simulink model "ex6_aberta"  (Simulink 8.9)
settings: Solver=FixedStepAuto  StartTime=0.0  StopTime=4  FixedStep=0.00442  RelTol=1e-3  EnableMultiTasking=on
values from neighbouring files (symbols this model uses):
  c1 = 2.94    [exp01e03.m]
  k1 = 338.6    [exp01e03.m]
  khw = 14732    [exp01e03.m]
  kpfA = 1 / Gps0    [exp01e03.m]
  kv = 0.005    [exp01e03.m]
  m1 = mc1 + mw1    (= 2.778)    [exp01e03.m]
settings Model: Creator=Gabriel  LastModifiedBy=Gabriel
settings DataIOCC: LimitDataPoints=off
settings OptimizationCC: InitFltsAndDblsToZero=on
settings DebuggingCC: SaveWithParameterizedLinksMsg=none  SignalResolutionControl=TryResolveAllWithWarning  SolverPrmCheckMsg=warning  MultiTaskDSMMsg=warning  MultiTaskCondExecSysMsg=none  StateNameClashWarn=none
settings GRTTargetCC: TargetFcnLib=ansi_tfl_tmw.mat  GeneratePreprocessorConditionals=Use local settings

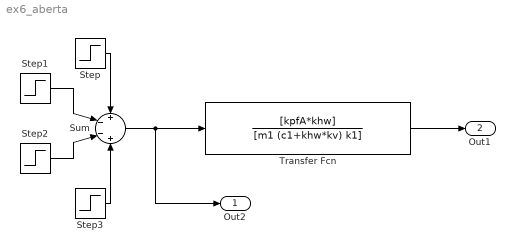
== system ex6_aberta ==
  Step : Step  Time=0  After=3000  SampleTime=0
  Step1 : Step  After=3000  SampleTime=0
  Step2 : Step  Time=2  After=3000  SampleTime=0
  Step3 : Step  Time=3  After=3000  SampleTime=0
  Sum : Sum  Inputs=+--+
  Transfer Fcn : TransferFcn  Numerator=[kpfA*khw]  Denominator=[m1 (c1+khw*kv) k1]
  Out2 : Outport
  Out1 : Outport  Port=2
  wires:
  Step/1 -> Sum/1
  Step1/1 -> Sum/2
  Step3/1 -> Sum/4
  Step2/1 -> Sum/3
  Sum/1 -> Out2/1, Transfer Fcn/1
  Transfer Fcn/1 -> Out1/1
